simulink model "araba_new"  (R2020a)
settings: Solver=VariableStepAuto  StartTime=0.0  StopTime=10.0  MaxStep=0.001  RelTol=1e-3
InitFcn:
  | kp = 0.35;
  | kc = 2;
  | l = 0.75;
  | g = 9.81;
  | f =2;
settings Model: Creator=muham  LastModifiedBy=muham

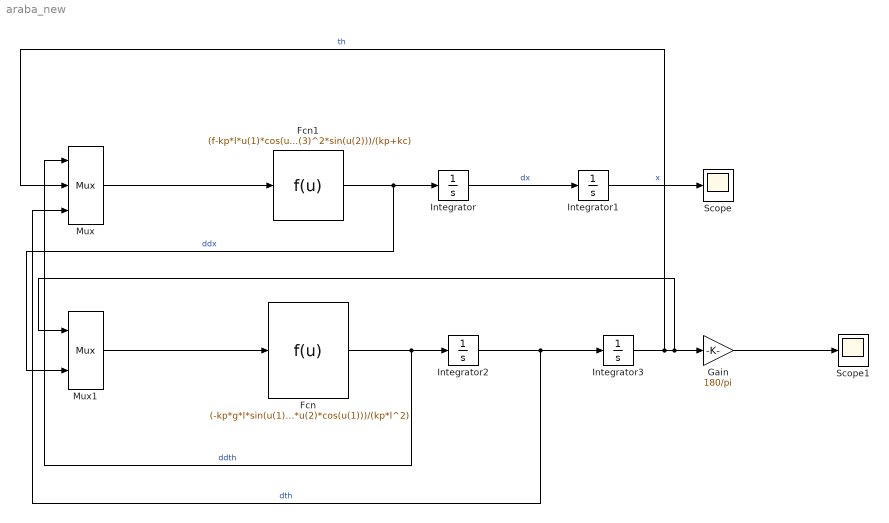
== system araba_new ==
  Fcn : Fcn  Expr=(-kp*g*l*sin(u(1))-kp*l*u(2)*cos(u(1)))/(kp*l^2)
  Fcn1 : Fcn  Expr=(f-kp*l*u(1)*cos(u(2))+kp*l*u(3)^2*sin(u(2)))/(kp+kc)
  Gain : Gain  Gain=180/pi
  Integrator : Integrator
  Integrator1 : Integrator  InitialCondition=0.5
  Integrator2 : Integrator
  Integrator3 : Integrator  InitialCondition=pi/3
  Mux : Mux  Inputs=3
  Mux1 : Mux  Inputs=2
  Scope : Scope
  Scope1 : Scope
  wires:
  Mux/1 -> Fcn1/1
  Mux1/1 -> Fcn/1
  Fcn1/1 -> Mux1/2, Integrator/1  "ddx"
  Integrator/1 -> Integrator1/1  "dx"
  Fcn/1 -> Mux/1, Integrator2/1  "ddth"
  Integrator2/1 -> Mux/3, Integrator3/1  "dth"
  Integrator1/1 -> Scope/1  "x"
  Integrator3/1 -> Mux/2, Mux1/1, Gain/1  "th"
  Gain/1 -> Scope1/1
